simulink model "IndustrialMicrogrid"  (R2023a)
settings: Solver=FixedStepDiscrete  StartTime=0.0  StopTime=10  FixedStep=Ts  RelTol=1e-3
PostLoadFcn:
  | IndustrialMicrogridInputData
  | GfmGridFormingConverterInputParameters
model workspace (MAT data in the model file):
  caseNum = 2
undefined symbols (not defined in the file): base, BESS, DiscIntNeverNeededParam, grid, Grid, gridInverter, machine, microgrid, PV, PVInverter, PVTransformer, scrFactorRg, scrFactorXg, transformer, Ts
libraries: ee_lib x112, eeGeneralControl x104, nesl_utility_internal x64, simulink x56, nesl_utility x37, fl_lib x29, slpidlib x13, eeTransforms x11, eeTotalHarmonicDistorsion x8, eeRmsMeasurement x4, eeSinusoidalMeasurement x4, simulink_extras x2
(part 7 of 14)

== system IndustrialMicrogrid/MG1 Primary Substation/Microgrid Controller/Planned Island/Control for Zero Powerflow ==
  Bus Element In{,1..4} (5 alike) : Inport  PortName=ControlRoom  Element=PlannedIslandCmd
  In Bus Element1 : Inport  Port=2  PortName=mPCCPLL  Element=PCC.mPCC.reactivepower
  In Bus Element7 : Inport  Port=2  PortName=mPCCPLL  Element=PCC.mPCC.activepower
  Logical Operator : Logic  AllPortsSameDT=off  OutDataTypeStr=boolean
  PID Frequency : slpidlib/PID Controller  Controller=PI  Form=Parallel  TimeDomain=Discrete-time  UseExternalTs=off  SampleTime=2*Ts  IntegratorMethod=Forward Euler  FilterMethod=Forward Euler  ControllerParametersSource=internal  P=KpPPlannedIsland  I=KiPPlannedIsland  UseKiTs=off  D=0  N=100  UseFilter=on  TunerSelectOption=Frequency Response Based  InitialConditionSource=internal  InitialConditionForIntegrator=0  InitialConditionForFilter=0  DifferentiatorICPrevScaledInput=0  ExternalReset=none  TrackingMode=off  Kt=1  LimitOutput=off  SatLimitsSource=internal  UpperSaturationLimit=0.05  LowerSaturationLimit=-0.05  LinearizeAsGain=on  AntiWindupMode=clamping  Kb=1  LimitIntegrator=off  UpperIntegratorSaturationLimit=inf  LowerIntegratorSaturationLimit=-inf  POutMin=[]  POutMax=[]  IOutMin=[]  IOutMax=[]  DOutMin=[]  DOutMax=[]  NOutMin=[]  NOutMax=[]  SumOutMin=[]  SumOutMax=[]  SaturationOutMin=[]  SaturationOutMax=[]  PParamMin=[]  PParamMax=[]  IParamMin=[]  IParamMax=[]  DParamMin=[]  DParamMax=[]  NParamMin=[]  NParamMax=[]  KbParamMin=[]  KbParamMax=[]  KtParamMin=[]  KtParamMax=[]  KbOutMin=[]  KbOutMax=[]  KtOutMin=[]  KtOutMax=[]  IntegratorOutMin=[]  IntegratorOutMax=[]  FilterOutMin=[]  FilterOutMax=[]  SumI1OutMin=[]  SumI1OutMax=[]  SumI2OutMin=[]  SumI2OutMax=[]  SumI3OutMin=[]  SumI3OutMax=[]  SumI4OutMin=[]  SumI4OutMax=[]  SumDOutMin=[]  SumDOutMax=[]  DifferentiatorOutMin=[]  DifferentiatorOutMax=[]  FilterDiffOutCoefMin=[]  FilterDiffOutCoefMax=[]  ReciprocalOutMin=[]  ReciprocalOutMax=[]  SumDenOutMin=[]  SumDenOutMax=[]  SumNumOutMin=[]  SumNumOutMax=[]  DivideOutMin=[]  DivideOutMax=[]  UdiffTsProdOutMin=[]  UdiffTsProdOutMax=[]  NTsProdOutMin=[]  NTsProdOutMax=[]  UintegralTsProdOutMin=[]  UintegralTsProdOutMax=[]  UngainTsProdOutMin=[]  UngainTsProdOutMax=[]  ClampingZeroOutDataTypeStr=Inherit: Inherit via back propagation  ClampingZeroOutMin=[]  ClampingZeroOutMax=[]  FilterDenConstantOutDataTypeStr=Inherit: Inherit via back propagation  FilterDenConstantOutMin=[]  FilterDenConstantOutMax=[]  PCopyOutDataTypeStr=Inherit: Inherit via back propagation  PCopyOutMin=[]  PCopyOutMax=[]  NCopyOutDataTypeStr=Inherit: Inherit via back propagation  NCopyOutMin=[]  NCopyOutMax=[]  IntegratorContinuousStateAttributes=''  IntegratorStateMustResolveToSignalObject=off  IntegratorRTWStateStorageClass=Auto  FilterContinuousStateAttributes=''  FilterStateMustResolveToSignalObject=off  FilterRTWStateStorageClass=Auto  ParallelPVariant=InternalParameters  IdealPVariant=Disabled  IVariant=InternalParameters  DVariant=Disabled  IntegratorVariant=Discrete  SatVariant=Disabled  AWVariant=Passthrough  PCopyVariant=Disabled  TRVariant=Disabled  FdbkBlocksVariant=Forward  IdealPFdbkVariant=Disabled  SatFdbkVariant=Disabled  DerivativeFilterVariant=Disabled  NVariant=Disabled  NCopyVariant=Disabled_SignalSpec  FilterICVariant=Disabled  IntegratorICVariant=InternalICs  ExternalResetVariant=Disabled  TRSumVariant=Passthrough  SumFdbkVariant=Disabled  SumVariant=Sum_PI  TsampFilterVariant=InternalTs  TsampNgainVariant=Passthrough  TsampIntegralVariant=Disabled_SignalSpec  ExternalSaturationOutDataTypeStr=Inherit: Same as second input
  PID voltage : slpidlib/PID Controller  Controller=PI  Form=Parallel  TimeDomain=Discrete-time  UseExternalTs=off  SampleTime=2*Ts  IntegratorMethod=Forward Euler  FilterMethod=Forward Euler  ControllerParametersSource=internal  P=KpQPlannedIsland  I=KiQPlannedIsland  UseKiTs=off  D=0  N=100  UseFilter=on  TunerSelectOption=Frequency Response Based  InitialConditionSource=internal  InitialConditionForIntegrator=0  InitialConditionForFilter=0  DifferentiatorICPrevScaledInput=0  ExternalReset=none  TrackingMode=off  Kt=1  LimitOutput=off  SatLimitsSource=internal  UpperSaturationLimit=0.05  LowerSaturationLimit=-0.05  LinearizeAsGain=on  AntiWindupMode=clamping  Kb=1  LimitIntegrator=off  UpperIntegratorSaturationLimit=inf  LowerIntegratorSaturationLimit=-inf  POutMin=[]  POutMax=[]  IOutMin=[]  IOutMax=[]  DOutMin=[]  DOutMax=[]  NOutMin=[]  NOutMax=[]  SumOutMin=[]  SumOutMax=[]  SaturationOutMin=[]  SaturationOutMax=[]  PParamMin=[]  PParamMax=[]  IParamMin=[]  IParamMax=[]  DParamMin=[]  DParamMax=[]  NParamMin=[]  NParamMax=[]  KbParamMin=[]  KbParamMax=[]  KtParamMin=[]  KtParamMax=[]  KbOutMin=[]  KbOutMax=[]  KtOutMin=[]  KtOutMax=[]  IntegratorOutMin=[]  IntegratorOutMax=[]  FilterOutMin=[]  FilterOutMax=[]  SumI1OutMin=[]  SumI1OutMax=[]  SumI2OutMin=[]  SumI2OutMax=[]  SumI3OutMin=[]  SumI3OutMax=[]  SumI4OutMin=[]  SumI4OutMax=[]  SumDOutMin=[]  SumDOutMax=[]  DifferentiatorOutMin=[]  DifferentiatorOutMax=[]  FilterDiffOutCoefMin=[]  FilterDiffOutCoefMax=[]  ReciprocalOutMin=[]  ReciprocalOutMax=[]  SumDenOutMin=[]  SumDenOutMax=[]  SumNumOutMin=[]  SumNumOutMax=[]  DivideOutMin=[]  DivideOutMax=[]  UdiffTsProdOutMin=[]  UdiffTsProdOutMax=[]  NTsProdOutMin=[]  NTsProdOutMax=[]  UintegralTsProdOutMin=[]  UintegralTsProdOutMax=[]  UngainTsProdOutMin=[]  UngainTsProdOutMax=[]  ClampingZeroOutDataTypeStr=Inherit: Inherit via back propagation  ClampingZeroOutMin=[]  ClampingZeroOutMax=[]  FilterDenConstantOutDataTypeStr=Inherit: Inherit via back propagation  FilterDenConstantOutMin=[]  FilterDenConstantOutMax=[]  PCopyOutDataTypeStr=Inherit: Inherit via back propagation  PCopyOutMin=[]  PCopyOutMax=[]  NCopyOutDataTypeStr=Inherit: Inherit via back propagation  NCopyOutMin=[]  NCopyOutMax=[]  IntegratorContinuousStateAttributes=''  IntegratorStateMustResolveToSignalObject=off  IntegratorRTWStateStorageClass=Auto  FilterContinuousStateAttributes=''  FilterStateMustResolveToSignalObject=off  FilterRTWStateStorageClass=Auto  ParallelPVariant=InternalParameters  IdealPVariant=Disabled  IVariant=InternalParameters  DVariant=Disabled  IntegratorVariant=Discrete  SatVariant=Disabled  AWVariant=Passthrough  PCopyVariant=Disabled  TRVariant=Disabled  FdbkBlocksVariant=Forward  IdealPFdbkVariant=Disabled  SatFdbkVariant=Disabled  DerivativeFilterVariant=Disabled  NVariant=Disabled  NCopyVariant=Disabled_SignalSpec  FilterICVariant=Disabled  IntegratorICVariant=InternalICs  ExternalResetVariant=Disabled  TRSumVariant=Passthrough  SumFdbkVariant=Disabled  SumVariant=Sum_PI  TsampFilterVariant=InternalTs  TsampNgainVariant=Passthrough  TsampIntegralVariant=Disabled_SignalSpec  ExternalSaturationOutDataTypeStr=Inherit: Same as second input
  Planned Island Time Delay : Subsystem
  Product{,1..3} (4 alike) : Product
  Subsystem : Subsystem
  Subsystem1 : Subsystem
  Bus Element Out : Outport  PortName=MGController  Element=plannedisland
  Bus Element Out1 : Outport  PortName=MGController  Element=plannedislandP
  Bus Element Out2 : Outport  PortName=MGController  Element=plannedislandQ
  Bus Element Out4 : Outport  PortName=MGController  Element=activepowererror
  Bus Element Out6 : Outport  PortName=MGController  Element=reactivepowerrror
  wires:
  Logical Operator/1 -> Planned Island Time Delay/1(In1)
  Planned Island Time Delay/1(MGController) -> Bus Element Out/1
  Bus Element In3/1 -> Planned Island Time Delay/2(In2)
  PID voltage/1 -> Bus Element Out2/1  "REACTIVE POWER"
  Bus Element In2/1 -> Product2/2
  Bus Element In/1 -> Product1/2
  Product2/1 -> Subsystem1/1(REACTIVEPOWER ERROR), PID voltage/1, Bus Element Out6/1  "REACTIVEPOWER ERROR"
  Product1/1 -> PID Frequency/1, Bus Element Out4/1, Subsystem/1(AVTIVE POWER ERROR)  "AVTIVE POWER ERROR"
  PID Frequency/1 -> Bus Element Out1/1  "ACTIVE POWER"
  In Bus Element1/1 -> Product2/1
  In Bus Element7/1 -> Product1/1
  Bus Element In1/1 -> Product/1
  Product/1 -> Logical Operator/1
  Product3/1 -> Logical Operator/2
  Bus Element In4/1 -> Product3/1
  Subsystem/1(Out1) -> Product/2
  Subsystem1/1(Out1) -> Product3/2

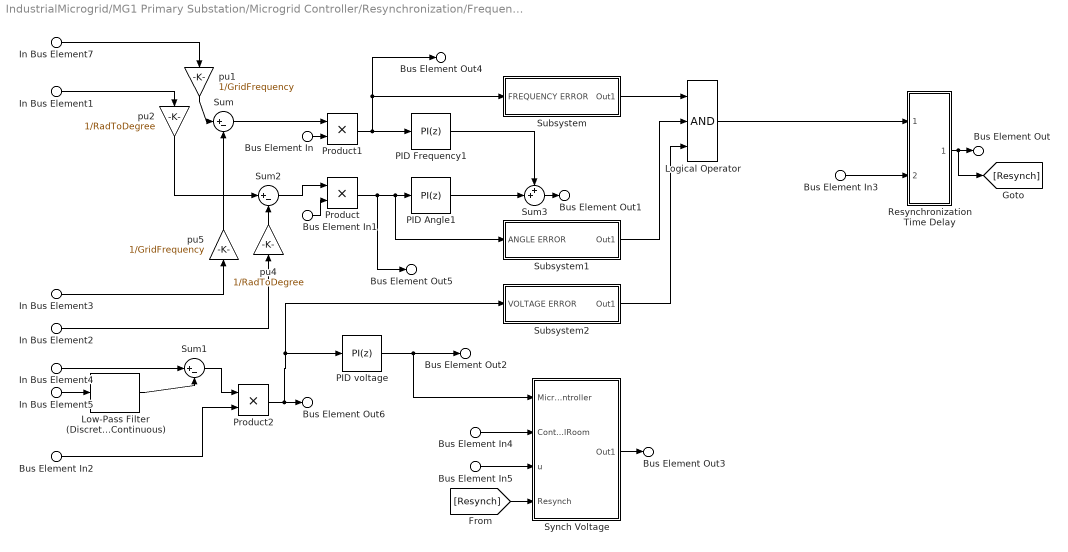
== system IndustrialMicrogrid/MG1 Primary Substation/Microgrid Controller/Resynchronization/Frequency and voltage matching ==
  Bus Element In5 : Inport  PortName=BESS  Element=reactive power
  Bus Element In{,1..4} (5 alike) : Inport  Port=2  PortName=ControlRoom  Element=ResynchCmd
  In Bus Element1 : Inport  Port=3  PortName=mPCCPLL  Element=Grid.angle
  In Bus Element7 : Inport  Port=3  PortName=mPCCPLL  Element=Grid.frequency
  In Bus Element4 : Inport  Port=3  PortName=mPCCPLL  Element=Grid.voltage
  In Bus Element3 : Inport  Port=3  PortName=mPCCPLL  Element=Island.frequency
  In Bus Element2 : Inport  Port=3  PortName=mPCCPLL  Element=Island.angle
  In Bus Element5 : Inport  Port=3  PortName=mPCCPLL  Element=Island.voltage
  Logical Operator : Logic  Inputs=3  AllPortsSameDT=off  OutDataTypeStr=boolean
  Low-Pass Filter (Discrete or Continuous) : eeGeneralControl/Low-Pass Filter (Discrete or Continuous)  K=1  T=0.04  B=inf  A=-inf  init_option=Inherited from block input  x0=0  Ts=-1
  PID Angle1 : slpidlib/PID Controller  Controller=PI  Form=Parallel  TimeDomain=Discrete-time  UseExternalTs=off  SampleTime=2*Ts  IntegratorMethod=Forward Euler  FilterMethod=Forward Euler  ControllerParametersSource=internal  P=KpAngResynch  I=KiAngResynch  UseKiTs=off  D=0  N=100  UseFilter=on  TunerSelectOption=Frequency Response Based  InitialConditionSource=internal  InitialConditionForIntegrator=0  InitialConditionForFilter=0  DifferentiatorICPrevScaledInput=0  ExternalReset=none  TrackingMode=off  Kt=1  LimitOutput=off  SatLimitsSource=internal  UpperSaturationLimit=0.05  LowerSaturationLimit=-0.05  LinearizeAsGain=on  AntiWindupMode=clamping  Kb=1  LimitIntegrator=off  UpperIntegratorSaturationLimit=inf  LowerIntegratorSaturationLimit=-inf  POutMin=[]  POutMax=[]  IOutMin=[]  IOutMax=[]  DOutMin=[]  DOutMax=[]  NOutMin=[]  NOutMax=[]  SumOutMin=[]  SumOutMax=[]  SaturationOutMin=[]  SaturationOutMax=[]  PParamMin=[]  PParamMax=[]  IParamMin=[]  IParamMax=[]  DParamMin=[]  DParamMax=[]  NParamMin=[]  NParamMax=[]  KbParamMin=[]  KbParamMax=[]  KtParamMin=[]  KtParamMax=[]  KbOutMin=[]  KbOutMax=[]  KtOutMin=[]  KtOutMax=[]  IntegratorOutMin=[]  IntegratorOutMax=[]  FilterOutMin=[]  FilterOutMax=[]  SumI1OutMin=[]  SumI1OutMax=[]  SumI2OutMin=[]  SumI2OutMax=[]  SumI3OutMin=[]  SumI3OutMax=[]  SumI4OutMin=[]  SumI4OutMax=[]  SumDOutMin=[]  SumDOutMax=[]  DifferentiatorOutMin=[]  DifferentiatorOutMax=[]  FilterDiffOutCoefMin=[]  FilterDiffOutCoefMax=[]  ReciprocalOutMin=[]  ReciprocalOutMax=[]  SumDenOutMin=[]  SumDenOutMax=[]  SumNumOutMin=[]  SumNumOutMax=[]  DivideOutMin=[]  DivideOutMax=[]  UdiffTsProdOutMin=[]  UdiffTsProdOutMax=[]  NTsProdOutMin=[]  NTsProdOutMax=[]  UintegralTsProdOutMin=[]  UintegralTsProdOutMax=[]  UngainTsProdOutMin=[]  UngainTsProdOutMax=[]  ClampingZeroOutDataTypeStr=Inherit: Inherit via back propagation  ClampingZeroOutMin=[]  ClampingZeroOutMax=[]  FilterDenConstantOutDataTypeStr=Inherit: Inherit via back propagation  FilterDenConstantOutMin=[]  FilterDenConstantOutMax=[]  PCopyOutDataTypeStr=Inherit: Inherit via back propagation  PCopyOutMin=[]  PCopyOutMax=[]  NCopyOutDataTypeStr=Inherit: Inherit via back propagation  NCopyOutMin=[]  NCopyOutMax=[]  IntegratorContinuousStateAttributes=''  IntegratorStateMustResolveToSignalObject=off  IntegratorRTWStateStorageClass=Auto  FilterContinuousStateAttributes=''  FilterStateMustResolveToSignalObject=off  FilterRTWStateStorageClass=Auto  ParallelPVariant=InternalParameters  IdealPVariant=Disabled  IVariant=InternalParameters  DVariant=Disabled  IntegratorVariant=Discrete  SatVariant=Disabled  AWVariant=Passthrough  PCopyVariant=Disabled  TRVariant=Disabled  FdbkBlocksVariant=Forward  IdealPFdbkVariant=Disabled  SatFdbkVariant=Disabled  DerivativeFilterVariant=Disabled  NVariant=Disabled  NCopyVariant=Disabled_SignalSpec  FilterICVariant=Disabled  IntegratorICVariant=InternalICs  ExternalResetVariant=Disabled  TRSumVariant=Passthrough  SumFdbkVariant=Disabled  SumVariant=Sum_PI  TsampFilterVariant=InternalTs  TsampNgainVariant=Passthrough  TsampIntegralVariant=Disabled_SignalSpec  ExternalSaturationOutDataTypeStr=Inherit: Same as second input
  PID Frequency1 : slpidlib/PID Controller  Controller=PI  Form=Parallel  TimeDomain=Discrete-time  UseExternalTs=off  SampleTime=2*Ts  IntegratorMethod=Forward Euler  FilterMethod=Forward Euler  ControllerParametersSource=internal  P=KpFreResynch  I=KiFreResynch  UseKiTs=off  D=0  N=100  UseFilter=on  TunerSelectOption=Frequency Response Based  InitialConditionSource=internal  InitialConditionForIntegrator=0  InitialConditionForFilter=0  DifferentiatorICPrevScaledInput=0  ExternalReset=none  TrackingMode=off  Kt=1  LimitOutput=off  SatLimitsSource=internal  UpperSaturationLimit=0.05  LowerSaturationLimit=-0.05  LinearizeAsGain=on  AntiWindupMode=clamping  Kb=1  LimitIntegrator=off  UpperIntegratorSaturationLimit=inf  LowerIntegratorSaturationLimit=-inf  POutMin=[]  POutMax=[]  IOutMin=[]  IOutMax=[]  DOutMin=[]  DOutMax=[]  NOutMin=[]  NOutMax=[]  SumOutMin=[]  SumOutMax=[]  SaturationOutMin=[]  SaturationOutMax=[]  PParamMin=[]  PParamMax=[]  IParamMin=[]  IParamMax=[]  DParamMin=[]  DParamMax=[]  NParamMin=[]  NParamMax=[]  KbParamMin=[]  KbParamMax=[]  KtParamMin=[]  KtParamMax=[]  KbOutMin=[]  KbOutMax=[]  KtOutMin=[]  KtOutMax=[]  IntegratorOutMin=[]  IntegratorOutMax=[]  FilterOutMin=[]  FilterOutMax=[]  SumI1OutMin=[]  SumI1OutMax=[]  SumI2OutMin=[]  SumI2OutMax=[]  SumI3OutMin=[]  SumI3OutMax=[]  SumI4OutMin=[]  SumI4OutMax=[]  SumDOutMin=[]  SumDOutMax=[]  DifferentiatorOutMin=[]  DifferentiatorOutMax=[]  FilterDiffOutCoefMin=[]  FilterDiffOutCoefMax=[]  ReciprocalOutMin=[]  ReciprocalOutMax=[]  SumDenOutMin=[]  SumDenOutMax=[]  SumNumOutMin=[]  SumNumOutMax=[]  DivideOutMin=[]  DivideOutMax=[]  UdiffTsProdOutMin=[]  UdiffTsProdOutMax=[]  NTsProdOutMin=[]  NTsProdOutMax=[]  UintegralTsProdOutMin=[]  UintegralTsProdOutMax=[]  UngainTsProdOutMin=[]  UngainTsProdOutMax=[]  ClampingZeroOutDataTypeStr=Inherit: Inherit via back propagation  ClampingZeroOutMin=[]  ClampingZeroOutMax=[]  FilterDenConstantOutDataTypeStr=Inherit: Inherit via back propagation  FilterDenConstantOutMin=[]  FilterDenConstantOutMax=[]  PCopyOutDataTypeStr=Inherit: Inherit via back propagation  PCopyOutMin=[]  PCopyOutMax=[]  NCopyOutDataTypeStr=Inherit: Inherit via back propagation  NCopyOutMin=[]  NCopyOutMax=[]  IntegratorContinuousStateAttributes=''  IntegratorStateMustResolveToSignalObject=off  IntegratorRTWStateStorageClass=Auto  FilterContinuousStateAttributes=''  FilterStateMustResolveToSignalObject=off  FilterRTWStateStorageClass=Auto  ParallelPVariant=InternalParameters  IdealPVariant=Disabled  IVariant=InternalParameters  DVariant=Disabled  IntegratorVariant=Discrete  SatVariant=Disabled  AWVariant=Passthrough  PCopyVariant=Disabled  TRVariant=Disabled  FdbkBlocksVariant=Forward  IdealPFdbkVariant=Disabled  SatFdbkVariant=Disabled  DerivativeFilterVariant=Disabled  NVariant=Disabled  NCopyVariant=Disabled_SignalSpec  FilterICVariant=Disabled  IntegratorICVariant=InternalICs  ExternalResetVariant=Disabled  TRSumVariant=Passthrough  SumFdbkVariant=Disabled  SumVariant=Sum_PI  TsampFilterVariant=InternalTs  TsampNgainVariant=Passthrough  TsampIntegralVariant=Disabled_SignalSpec  ExternalSaturationOutDataTypeStr=Inherit: Same as second input
  PID voltage : slpidlib/PID Controller  Controller=PI  Form=Parallel  TimeDomain=Discrete-time  UseExternalTs=off  SampleTime=2*Ts  IntegratorMethod=Forward Euler  FilterMethod=Forward Euler  ControllerParametersSource=internal  P=KpVolResynch  I=KiVolResynch  UseKiTs=off  D=0  N=100  UseFilter=on  TunerSelectOption=Frequency Response Based  InitialConditionSource=internal  InitialConditionForIntegrator=1  InitialConditionForFilter=0  DifferentiatorICPrevScaledInput=0  ExternalReset=none  TrackingMode=off  Kt=1  LimitOutput=off  SatLimitsSource=internal  UpperSaturationLimit=0.05  LowerSaturationLimit=-0.05  LinearizeAsGain=on  AntiWindupMode=clamping  Kb=1  LimitIntegrator=off  UpperIntegratorSaturationLimit=inf  LowerIntegratorSaturationLimit=-inf  POutMin=[]  POutMax=[]  IOutMin=[]  IOutMax=[]  DOutMin=[]  DOutMax=[]  NOutMin=[]  NOutMax=[]  SumOutMin=[]  SumOutMax=[]  SaturationOutMin=[]  SaturationOutMax=[]  PParamMin=[]  PParamMax=[]  IParamMin=[]  IParamMax=[]  DParamMin=[]  DParamMax=[]  NParamMin=[]  NParamMax=[]  KbParamMin=[]  KbParamMax=[]  KtParamMin=[]  KtParamMax=[]  KbOutMin=[]  KbOutMax=[]  KtOutMin=[]  KtOutMax=[]  IntegratorOutMin=[]  IntegratorOutMax=[]  FilterOutMin=[]  FilterOutMax=[]  SumI1OutMin=[]  SumI1OutMax=[]  SumI2OutMin=[]  SumI2OutMax=[]  SumI3OutMin=[]  SumI3OutMax=[]  SumI4OutMin=[]  SumI4OutMax=[]  SumDOutMin=[]  SumDOutMax=[]  DifferentiatorOutMin=[]  DifferentiatorOutMax=[]  FilterDiffOutCoefMin=[]  FilterDiffOutCoefMax=[]  ReciprocalOutMin=[]  ReciprocalOutMax=[]  SumDenOutMin=[]  SumDenOutMax=[]  SumNumOutMin=[]  SumNumOutMax=[]  DivideOutMin=[]  DivideOutMax=[]  UdiffTsProdOutMin=[]  UdiffTsProdOutMax=[]  NTsProdOutMin=[]  NTsProdOutMax=[]  UintegralTsProdOutMin=[]  UintegralTsProdOutMax=[]  UngainTsProdOutMin=[]  UngainTsProdOutMax=[]  ClampingZeroOutDataTypeStr=Inherit: Inherit via back propagation  ClampingZeroOutMin=[]  ClampingZeroOutMax=[]  FilterDenConstantOutDataTypeStr=Inherit: Inherit via back propagation  FilterDenConstantOutMin=[]  FilterDenConstantOutMax=[]  PCopyOutDataTypeStr=Inherit: Inherit via back propagation  PCopyOutMin=[]  PCopyOutMax=[]  NCopyOutDataTypeStr=Inherit: Inherit via back propagation  NCopyOutMin=[]  NCopyOutMax=[]  IntegratorContinuousStateAttributes=''  IntegratorStateMustResolveToSignalObject=off  IntegratorRTWStateStorageClass=Auto  FilterContinuousStateAttributes=''  FilterStateMustResolveToSignalObject=off  FilterRTWStateStorageClass=Auto  ParallelPVariant=InternalParameters  IdealPVariant=Disabled  IVariant=InternalParameters  DVariant=Disabled  IntegratorVariant=Discrete  SatVariant=Disabled  AWVariant=Passthrough  PCopyVariant=Disabled  TRVariant=Disabled  FdbkBlocksVariant=Forward  IdealPFdbkVariant=Disabled  SatFdbkVariant=Disabled  DerivativeFilterVariant=Disabled  NVariant=Disabled  NCopyVariant=Disabled_SignalSpec  FilterICVariant=Disabled  IntegratorICVariant=InternalICs  ExternalResetVariant=Disabled  TRSumVariant=Passthrough  SumFdbkVariant=Disabled  SumVariant=Sum_PI  TsampFilterVariant=InternalTs  TsampNgainVariant=Passthrough  TsampIntegralVariant=Disabled_SignalSpec  ExternalSaturationOutDataTypeStr=Inherit: Same as second input
  Product : Product
  Product1 : Product
  Product2 : Product
  Resynchronization Time Delay : Subsystem
  Subsystem : Subsystem
  Subsystem1 : Subsystem
  Subsystem2 : Subsystem
  Sum : Sum  Inputs=|+-
  Sum1 : Sum  Inputs=|+-
  Sum2 : Sum  Inputs=|+-
  Sum3 : Sum  Inputs=++|
  Synch Voltage : Subsystem
  pu1 : Gain  Gain=1/GridFrequency
  pu2 : Gain  Gain=1/RadToDegree
  pu4 : Gain  Gain=1/RadToDegree
  pu5 : Gain  Gain=1/GridFrequency
  Bus Element Out : Outport  PortName=MGController  Element=resynch
  Bus Element Out1 : Outport  PortName=MGController  Element=synchfrequency
  Bus Element Out2 : Outport  PortName=MGController  Element=synchvoltage
  Bus Element Out3 : Outport  PortName=MGController  Element=synchvoltagedpr
  Bus Element Out4 : Outport  PortName=MGController  Element=frequencyerror
  Bus Element Out5 : Outport  PortName=MGController  Element=phaseerror
  Bus Element Out6 : Outport  PortName=MGController  Element=voltagemagerror
  wires:
  Sum/1 -> Product1/1
  pu1/1 -> Sum/1
  pu4/1 -> Sum2/2
  pu2/1 -> Sum2/1
  pu5/1 -> Sum/2
  In Bus Element2/1 -> pu4/1
  In Bus Element3/1 -> pu5/1
  Sum1/1 -> Product2/1
  Subsystem/1(Out1) -> Logical Operator/1
  Subsystem1/1(Out1) -> Logical Operator/2
  Subsystem2/1(Out1) -> Logical Operator/3
  Sum3/1 -> Bus Element Out1/1
  PID Frequency1/1 -> Sum3/1
  PID Angle1/1 -> Sum3/2
  Sum2/1 -> Product/1
  Product/1 -> Bus Element Out5/1, Subsystem1/1(ANGLE ERROR), PID Angle1/1
  Product1/1 -> Bus Element Out4/1, Subsystem/1(FREQUENCY ERROR), PID Frequency1/1
  Product2/1 -> Subsystem2/1(VOLTAGE ERROR), PID voltage/1, Bus Element Out6/1
  Bus Element In/1 -> Product1/2
  Bus Element In1/1 -> Product/2
  Bus Element In2/1 -> Product2/2
  In Bus Element7/1 -> pu1/1
  In Bus Element1/1 -> pu2/1
  In Bus Element4/1 -> Sum1/1
  In Bus Element5/1 -> Low-Pass Filter (Discrete or Continuous)/1
  PID voltage/1 -> Bus Element Out2/1, Synch Voltage/1(MicrogridController)
  Bus Element In3/1 -> Resynchronization Time Delay/2(In2)
  Resynchronization Time Delay/1(MGController) -> [Resynch], Bus Element Out/1
  Logical Operator/1 -> Resynchronization Time Delay/1(In1)
  Bus Element In4/1 -> Synch Voltage/2(ControlRoom)
  Bus Element In5/1 -> Synch Voltage/3(u)
  Synch Voltage/1(Out1) -> Bus Element Out3/1
  [Resynch] -> Synch Voltage/4(Resynch)
  Low-Pass Filter (Discrete or Continuous)/1 -> Sum1/2

== system IndustrialMicrogrid/MG2 PV Plant/(500KWp PV)/PV Inverter A2/PV & Inverter ==
  note: Calculated PV power output
  note: Measured PV current
  note: Perturb & Observe method for maximum power point (MPP) tracking of PV array
  note: DC bus voltage reference (which is the MPP voltage)
  Solar insolation : Inport
  reference : Inport  Port=2
  Average-Inverter : ee_lib/Semiconductors & Converters/Converters/Average-Value Voltage Source Converter (Three-Phase)  port_option=ee.enum.threePhasePort.composite  frequency_option=ee.enum.converters.frequency.variable  FRated=60 Hz  losses_parameterization=ee.enum.converters.losses.fixed  Pfixed=1 W  ks=0.01  kc1=1.7 V  kc2=0.01 Ohm  Ploss_vect=[100, 800, 1870, 3250, 4900] W  Irms_vect=[10, 100, 200, 300, 400] A  Vdc_nom=300 V  thermal_mass=30000 J/K  temperature_specify=off  temperature_priority=High  temperature=298.15 K  temperature_nominal_specify=off  temperature_nominal_unit=K  temperature_nominal_value=1
      settings: InternalSimscapePortConfiguration="{\"Bottom\":[],\"Left\":[{\"id\":\"ModWave\",\"label\":\"ModWave\",\"type\":\"input\"},{\"id\":\"N\",\"label\":\"~\",\"type\":\"foundation.electrical.three_phase\"}],\"Right\":[{\"id\":\"p\",\"label\":\"+\",\"type\":\"foundation.electrical.electrical\"},{\"id\":\"n\",\"label\":\"-\",\"type\":\"foundation.electrical.electrical\"}],\"Top\":[]}"
  Current Sensor : fl_lib/Electrical/Electrical Sensors/Current Sensor
  DC- Capacitor : fl_lib/Electrical/Electrical Elements/Capacitor  c=PVInverter.c F  r=1e-6 Ohm  g=0 1/Ohm  i_specify=off  i_priority=None  i=0 A  i_nominal_specify=off  i_nominal_unit=A  i_nominal_value=1  v_specify=off  v_priority=None  v=6560*.5 V  v_nominal_specify=off  v_nominal_unit=V  v_nominal_value=1  vc_specify=on  vc_priority=None  vc=PVInverter.Vdc V  vc_nominal_specify=off  vc_nominal_unit=V  vc_nominal_value=1
  ERef1 : fl_lib/Electrical/Electrical Elements/Electrical Reference
  Low-Pass Filter (Discrete or Continuous) : eeGeneralControl/Low-Pass Filter (Discrete or Continuous)  K=1  T=0.2  B=inf  A=-inf  init_option=Inherited from block input  x0=0  Ts=-1
  Low-Pass Filter (Discrete or Continuous)1 : eeGeneralControl/Low-Pass Filter (Discrete or Continuous)  K=1  T=0.2  B=inf  A=-inf  init_option=Inherited from block input  x0=0  Ts=-1
  Measurement1 : Subsystem
  Measurement2 : Subsystem
  P&O MPP : Subsystem
  PS-Simulink Converter : nesl_utility/PS-Simulink Converter  PhysicalDomain=network_engine_domain  SubClassName=ps_output  LeftPortType=input  RightPortType=output  PseudoPeriodic=off  Frequencies=[]  VectorFormat=inherit  Unit=inherit  AffineConversion=off
  PS-Simulink Converter1 : nesl_utility/PS-Simulink Converter  PhysicalDomain=network_engine_domain  SubClassName=ps_output  LeftPortType=input  RightPortType=output  PseudoPeriodic=off  Frequencies=[]  VectorFormat=inherit  Unit=inherit  AffineConversion=off
  PV Array : ee_lib/Sources/Solar Cell  prm=3  Isc=3.8 A  Voc=0.586 V  Is=PV.solarCellDiodeSaturationCurrent A  Is2=0 A  Iph=PV.solarCellSolarGeneratedCurrentAM A  Ir0=1000 W/m^2  ec=PV.solarCellQualityFactorI  N2=PV.solarCellQualityFactorJ  Rs=PV.solarCellSeriesResistance Ohm  Rp=PV.solarCellParallelResistance Ohm  N_series=PV.panelNSeriesCellPanel*PV.arrayNseriesPanelsPerString  N_parallel=PV.PanelNParallelStringsPanel*PV.arrayNParallelStrings  TIPH1=PV.solarCellTempCofficient 1/K  EG=PV.solarCellEg eV  TXIS1=PV.solarCellTemparatureExponentIs1  TXIS2=PV.solarCellTemparatureExponentIs2  TRS1=PV.solarCellTemparatureExponentRs  TRP1=PV.solarCellTemparatureExponentRp  Tmeas=PV.solarCellMeasurementTemperature degC  TFIXED=PV.solarCellDeviceTemperature degC  thermal_mass=100 J/K  initial_temperature=25 degC
  Product2 : Product
  Simulink-PS Converter1 : nesl_utility/Simulink-PS Converter  PhysicalDomain=network_engine_domain  SubClassName=ps_input  LeftPortType=input  RightPortType=output  PseudoPeriodic=off  Frequencies=[]  NoiseDistribution=none  NoiseParameters=[]  Unit=1  AffineConversion=off  FilteringAndDerivatives=provide  SimscapeFilterOrder=1  InputFilterTimeConstant=0.001  UdotUserProvided=0
  Simulink-PS Converter2 : nesl_utility/Simulink-PS Converter  PhysicalDomain=network_engine_domain  SubClassName=ps_input  LeftPortType=input  RightPortType=output  PseudoPeriodic=off  Frequencies=[]  NoiseDistribution=none  NoiseParameters=[]  Unit=1  AffineConversion=off  FilteringAndDerivatives=provide  SimscapeFilterOrder=1  InputFilterTimeConstant=0.001  UdotUserProvided=0
  Voltage Sensor : fl_lib/Electrical/Electrical Sensors/Voltage Sensor
  Conn1 : PMIOPort  Side=Right
  Out Bus Element4 : Outport  PortName=PV_plant1  Element=Vdc_ref
  Out Bus Element : Outport  PortName=PV_plant1  Element=Pref1
  Out Bus Element3 : Outport  PortName=PV_plant1  Element=Vdc_measured
  Out Bus Element1 : Outport  PortName=PV_plant1  Element=ipv
  wires:
  Low-Pass Filter (Discrete or Continuous)1/1 -> Product2/2
  Low-Pass Filter (Discrete or Continuous)/1 -> [Vdc]
  Measurement2/1(Out1) -> [ipv]
  Measurement1/1(Out1) -> Low-Pass Filter (Discrete or Continuous)/1
  [Vdc] -> P&O MPP/2(Input)
  P&O MPP/1(Vmpp) -> Out Bus Element4/1
  Product2/1 -> Out Bus Element/1, P&O MPP/1(In1)
  reference/1 -> Simulink-PS Converter2/1
  [Vdc] -> Product2/1
  PS-Simulink Converter/1 -> Out Bus Element3/1, Measurement1/1(u)
  [ipv] -> Low-Pass Filter (Discrete or Continuous)1/1
  Solar insolation/1 -> Simulink-PS Converter1/1
  PS-Simulink Converter1/1 -> Out Bus Element1/1, Measurement2/1(u)
  connections:
  PV Array/RConn1 -- ERef1/LConn1 -- DC- Capacitor/RConn1 -- Average-Inverter/RConn2 -- Voltage Sensor/RConn2
  Simulink-PS Converter1/RConn1 -- PV Array/LConn1
  PS-Simulink Converter1/LConn1 -- Current Sensor/RConn1
  Conn1/RConn1 -- Average-Inverter/LConn2
  PV Array/LConn2 -- Current Sensor/LConn1
  Average-Inverter/LConn1 -- Simulink-PS Converter2/RConn1
  Voltage Sensor/LConn1 -- Current Sensor/RConn2 -- Average-Inverter/RConn1 -- DC- Capacitor/LConn1
  PS-Simulink Converter/LConn1 -- Voltage Sensor/RConn1

== system IndustrialMicrogrid/MG2 PV Plant/(500KWp PV)/PV Inverter A2/PV Controller ==
  note: DQ/abc Transformation
  In Bus Element17 : Inport  PortName=PV_plant1  Element=Pref1
  In Bus Element18 : Inport  PortName=PV_plant1  Element=Vdc_measured
  In Bus Element19 : Inport  PortName=PV_plant1  Element=Vdc_ref
  In Bus Element5 : Inport  Port=2  PortName=ipv1  Element=1
  In Bus Element4 : Inport  Port=3  PortName=LVRT
  In Bus Element3 : Inport  Port=4  PortName=Vbus  Element=Vd
  In Bus Element1 : Inport  Port=4  PortName=Vbus  Element=Vd
  In Bus Element2 : Inport  Port=4  PortName=Vbus  Element=Vq
  In Bus Element6 : Inport  Port=4  PortName=Vbus  Element=Theta
  In Bus Element7 : Inport  Port=4  PortName=Vbus  Element=Theta
  Q_ref : Inport  Port=5
  Current_controller : Subsystem
  DC voltage controller & current reference : Subsystem
  Demux1 : Demux  Outputs=3
  Inverse Park Transform1 : eeTransforms/Inverse Park Transform  AxisAlignment=Q-axis  PowerInvariant=off
  Park Transform1 : eeTransforms/Park Transform  AxisAlignment=Q-axis  PowerInvariant=off
  Terminator1 : Terminator
  Unit Delay2 : UnitDelay  SampleTime=Ts  HasFrameUpgradeWarning=on
  m_abc : Outport
  wires:
  Q_ref/1 -> DC voltage controller & current reference/1(Q_ref)
  DC voltage controller & current reference/2(id_ref) -> [id_ref]
  DC voltage controller & current reference/1(iq_ref) -> [iq_ref]
  In Bus Element19/1 -> DC voltage controller & current reference/5(PV_vdc)
  In Bus Element18/1 -> DC voltage controller & current reference/4(PV_Mpp_vdc)
  In Bus Element17/1 -> DC voltage controller & current reference/3(P_pv)
  In Bus Element4/1 -> DC voltage controller & current reference/6(LVRT.iq)
  In Bus Element1/1 -> DC voltage controller & current reference/2(Vmag)
  In Bus Element5/1 -> Park Transform1/1
  [ipvd] -> Current_controller/2(ipvd)
  In Bus Element7/1 -> Inverse Park Transform1/2
  In Bus Element6/1 -> Park Transform1/2
  [ipvq] -> Current_controller/4(iq)
  [iq_ref] -> Current_controller/3(iqref)
  In Bus Element3/1 -> Current_controller/5(Vd)
  [id_ref] -> Current_controller/1(id-ref)
  Park Transform1/1 -> Demux1/1
  [mdqo] -> Inverse Park Transform1/1
  Demux1/3 -> Terminator1/1
  Demux1/1 -> [ipvd]
  Unit Delay2/1 -> m_abc/1
  Demux1/2 -> [ipvq]
  Inverse Park Transform1/1 -> Unit Delay2/1
  Current_controller/1(Refrence_mdq0) -> [mdqo]
  In Bus Element2/1 -> Current_controller/6(Vq)

== system IndustrialMicrogrid/MG2 Power Center/Diesel Generator/Governor and Prime Mover /Governor ==
  pu_velocity : Inport
  1/T_G : Gain  Gain=1/T_G
  1/droop : Gain  Gain=1/(droop_percentage/100)
  Delta load setpoint : Sum  Inputs=+-|
  Delta speed : Sum  Inputs=-+|
  Discrete-Time Integrator1 : DiscreteIntegrator  InitialCondition=pu_torque0  SampleTime=-1  ICPrevOutput=DiscIntNeverNeededParam  ICPrevScaledInput=DiscIntNeverNeededParam
  Load_setpoint : Constant  Value=pu_load_reference_setpoint
  Speed_ref : Constant  Value=pu_speed_reference
  Subtract : Sum  Inputs=|+-
  delta_y : Outport  VectorParamsAs1DForOutWhenUnconnected=off
  wires:
  Speed_ref/1 -> Delta speed/1
  Delta speed/1 -> 1/droop/1
  Load_setpoint/1 -> Delta load setpoint/1
  pu_velocity/1 -> Delta speed/2
  1/droop/1 -> Delta load setpoint/2
  Delta load setpoint/1 -> Subtract/1
  Subtract/1 -> 1/T_G/1
  1/T_G/1 -> Discrete-Time Integrator1/1
  Discrete-Time Integrator1/1 -> delta_y/1, Subtract/2

== system IndustrialMicrogrid/MG2 Power Center/Diesel Generator/Governor and Prime Mover /Non-reheat turbine ==
  delta_y : Inport
  1/T_CH : Gain  Gain=1/T_CH
  Discrete-Time Integrator1 : DiscreteIntegrator  InitialCondition=pu_torque0  SampleTime=-1  ICPrevOutput=DiscIntNeverNeededParam  ICPrevScaledInput=DiscIntNeverNeededParam
  Sum : Sum  Inputs=|+-
  torque : Outport  VectorParamsAs1DForOutWhenUnconnected=off
  wires:
  delta_y/1 -> Sum/1
  Sum/1 -> 1/T_CH/1
  1/T_CH/1 -> Discrete-Time Integrator1/1
  Discrete-Time Integrator1/1 -> Sum/2, torque/1

== system IndustrialMicrogrid/MG2 Primary Substation/BESS and Controller 2/BESS/Filter & Sensor ==
  Current Sensor (Three-Phase) : ee_lib/Sensors & Transducers/Current Sensor (Three-Phase)
  Electrical Reference1 : fl_lib/Electrical/Electrical Elements/Electrical Reference
  Low-Pass Filter (Discrete or Continuous)1 : eeGeneralControl/Low-Pass Filter (Discrete or Continuous)  K=1  T=1/(200*gridInverter.frequency)  B=inf  A=-inf  init_option=Specify as parameter  x0=0  Ts=gridInverter.controller.VoltageControlSampleTime
  Low-Pass Filter (Discrete or Continuous)2 : eeGeneralControl/Low-Pass Filter (Discrete or Continuous)  K=1  T=1/(200*gridInverter.frequency)  B=inf  A=-inf  init_option=Specify as parameter  x0=0  Ts=gridInverter.controller.VoltageControlSampleTime
  Neutral Port (Three-Phase) : ee_lib/Connectors & References/Neutral Port (Three-Phase)  G_parasitic=1e-12 1/Ohm
      settings: InternalSimscapePortConfiguration="{\"Bottom\":[],\"Left\":[{\"id\":\"N\",\"label\":\"~\",\"type\":\"foundation.electrical.three_phase\"}],\"Right\":[{\"id\":\"n\",\"label\":\"n\",\"type\":\"foundation.electrical.electrical\"}],\"Top\":[]}"
  PS-Simulink Converter : nesl_utility/PS-Simulink Converter  PhysicalDomain=network_engine_domain  SubClassName=ps_output  LeftPortType=input  RightPortType=output  PseudoPeriodic=off  Frequencies=[]  VectorFormat=inherit  Unit=inherit  AffineConversion=off
  PS-Simulink Converter1 : nesl_utility/PS-Simulink Converter  PhysicalDomain=network_engine_domain  SubClassName=ps_output  LeftPortType=input  RightPortType=output  PseudoPeriodic=off  Frequencies=[]  VectorFormat=inherit  Unit=inherit  AffineConversion=off
  Phase Voltage Sensor (Three-Phase) : ee_lib/Sensors & Transducers/Phase Voltage Sensor (Three-Phase)
  RLC (Three-Phase) : ee_lib/Passive/RLC Assemblies/RLC (Three-Phase)  component_structure=ee.enum.rlc.structure.SeriesRL  R=gridInverter.lineResistance Ohm  L=gridInverter.L*10 H  C=1e-6 F  R_parasitic=0 Ohm  G_parasitic=0 1/Ohm  IL_specify=off  IL_priority=High  IL=[0, 0, 0] A  IL_nominal_specify=off  IL_nominal_unit=A  IL_nominal_value=1  VC_specify=off  VC_priority=High  VC=[0, 0, 0] V  VC_nominal_specify=off  VC_nominal_unit=V  VC_nominal_value=1
      settings: InternalSimscapePortConfiguration="{\"Bottom\":[],\"Left\":[{\"id\":\"N1\",\"label\":\"~1\",\"type\":\"foundation.electrical.three_phase\"}],\"Right\":[{\"id\":\"N2\",\"label\":\"~2\",\"type\":\"foundation.electrical.three_phase\"}],\"Top\":[]}"
  Inabc : PMIOPort  Side=Left
  Opabc : PMIOPort  Port=2  Side=Right
  Iabc : Outport
  Vabc : Outport  Port=2
  wires:
  PS-Simulink Converter1/1 -> Low-Pass Filter (Discrete or Continuous)1/1
  Low-Pass Filter (Discrete or Continuous)2/1 -> Iabc/1
  PS-Simulink Converter/1 -> Low-Pass Filter (Discrete or Continuous)2/1
  Low-Pass Filter (Discrete or Continuous)1/1 -> Vabc/1
  connections:
  Electrical Reference1/LConn1 -- Neutral Port (Three-Phase)/RConn1
  PS-Simulink Converter1/LConn1 -- Phase Voltage Sensor (Three-Phase)/RConn1
  Current Sensor (Three-Phase)/RConn2 -- RLC (Three-Phase)/LConn1
  Neutral Port (Three-Phase)/LConn1 -- Phase Voltage Sensor (Three-Phase)/RConn2
  Current Sensor (Three-Phase)/LConn1 -- Inabc/RConn1
  PS-Simulink Converter/LConn1 -- Current Sensor (Three-Phase)/RConn1
  Phase Voltage Sensor (Three-Phase)/LConn1 -- Opabc/RConn1 -- RLC (Three-Phase)/RConn1

== system IndustrialMicrogrid/MG2 Primary Substation/BESS and Controller 2/BESS/Grid-Forming Converter Control ==
  Pref : Inport
  Qref : Inport  Port=2
  Vref : Inport  Port=3
  Fref : Inport  Port=4
  CntrlFlag : Inport  Port=5
  Igabc : Inport  Port=6
  Vgabc : Inport  Port=7
  BlackStart : Inport  Port=8
  Current Limiting : Subsystem
  Grid Voltage Reactive Power Support : Subsystem
  Measurement : Subsystem
      mask Display: image('$imagefile'); % Use "Edit Image" on toolstrip to change.
  Power Control : Subsystem
  VoltageCurrentControl : Subsystem
      settings: PortSchema="{\"entries\":[{\"content\":{\"sides\":[{\"content\":{\"connectorIds\":[\"In1\",\"In2\",\"In3\"]},\"type\":\"ConnectorPlacement.EquallySpacedRectSide\",\"uuid\":\"0bf15a12-7bc0-47e4-89bd-435769673763\"},{\"content\":{\"connectorIds\":[\"Out1\"],\"side\":\"RIGHT\"},\"type\":\"ConnectorPlacement.EquallySpacedRectSide\",\"uuid\":\"44a15d74-8878-4ec6-abe4-be0b1b609519\"},{\"content\":{\"connectorIds\":[\"In4\"],\"side\":\"TOP\"},\"type\":\"ConnectorPlacement.EquallySpacedRectSide\",\"uuid\":\"7a96781e-5638-4b2a-8101-d5785aae9f0f\"}]},\"type\":\"ConnectorPlacement.EquallySpacedConnector\",\"uuid\":\"4b3373ad-cf20-4175-894e-3bd1604dd0ce\"}],\"packageUris\":[\"http://schema.mathworks.com/mf0/Connector/R2020b\"],\"version\":\"1.0\"}"
  mabc : Outport
  Pmeas : Outport  Port=2
  Qmeas : Outport  Port=3
  fmeas : Outport  Port=4
  wires:
  VoltageCurrentControl/1(mabc) -> mabc/1
  Vgabc/1 -> Measurement/1(Vgabcc)
  Igabc/1 -> Measurement/2(Igabc)
  Measurement/2(Pmeas) -> Pmeas/1
  Measurement/3(Qmeas) -> Qmeas/1
  Measurement/1(measure) -> Current Limiting/1(measure), VoltageCurrentControl/4(measure), Power Control/1(measure), Grid Voltage Reactive Power Support/1(measure)
  Power Control/3(angle) -> Measurement/3(Angle)
  Power Control/1(reactiveControl) -> Current Limiting/2(reactiveControl)
  Power Control/2(activeControl) -> VoltageCurrentControl/2(activeControl)
  Current Limiting/1(currentLimiting) -> VoltageCurrentControl/1(currentLimiting)
  Qref/1 -> Grid Voltage Reactive Power Support/3(QrefInput)
  Pref/1 -> Grid Voltage Reactive Power Support/2(PrefInput)
  Grid Voltage Reactive Power Support/1(Pref) -> Power Control/2(Pref)
  Grid Voltage Reactive Power Support/2(Qref) -> Power Control/3(Qref)
  Measurement/4(fmeas) -> fmeas/1
  Fref/1 -> Power Control/5(Fref)
  Vref/1 -> Power Control/4(Vref)
  CntrlFlag/1 -> Power Control/6(CntrlFlag)
  BlackStart/1 -> VoltageCurrentControl/3(BlackStart)

== system IndustrialMicrogrid/MG2 Primary Substation/BESS and Controller 2/BESS/Per Unit Conversion ==
  fgrid : Inport
  Vabc : Inport  Port=2
  Iabc : Inport  Port=3
  Amp2PU : Gain  Gain=1/base.current
  PU2Hz : Gain  Gain=gridInverter.frequency
  Volt2PU : Gain  Gain=1/base.voltage
  fmeasHz : Outport
  Vabcpu : Outport  Port=2
  Iabcpu : Outport  Port=3
  wires:
  PU2Hz/1 -> fmeasHz/1
  fgrid/1 -> PU2Hz/1
  Volt2PU/1 -> Vabcpu/1  "Vabc"
  Iabc/1 -> Amp2PU/1
  Amp2PU/1 -> Iabcpu/1  "Iabc"
  Vabc/1 -> Volt2PU/1

== system IndustrialMicrogrid/MG2 Primary Substation/BESS and Controller 2/BESS/Subsystem ==
  PQref : Inport
  Demux : Demux  Outputs=2
  Low-Pass Filter (Discrete or Continuous) : eeGeneralControl/Low-Pass Filter (Discrete or Continuous)  K=1  T=5e-2  B=inf  A=-inf  init_option=Inherited from block input  x0=0  Ts=-1
  Low-Pass Filter (Discrete or Continuous)1 : eeGeneralControl/Low-Pass Filter (Discrete or Continuous)  K=1  T=5e-2  B=inf  A=-inf  init_option=Inherited from block input  x0=0  Ts=-1
  Unit Delay1 : UnitDelay  InitialCondition=1  SampleTime=Ts  HasFrameUpgradeWarning=on
  Unit Delay2 : UnitDelay  InitialCondition=1  SampleTime=Ts  HasFrameUpgradeWarning=on
  Pref : Outport
  Qref : Outport  Port=2
  wires:
  Demux/1 -> Unit Delay2/1  "Pref"
  Low-Pass Filter (Discrete or Continuous)/1 -> Pref/1
  Low-Pass Filter (Discrete or Continuous)1/1 -> Qref/1
  Demux/2 -> Unit Delay1/1  "Qref"
  PQref/1 -> Demux/1
  Unit Delay2/1 -> Low-Pass Filter (Discrete or Continuous)/1
  Unit Delay1/1 -> Low-Pass Filter (Discrete or Continuous)1/1

== system IndustrialMicrogrid/MG2 Primary Substation/BESS and Controller 2/BESS/Subsystem1 ==
  In1 : Inport
  Constant : Constant
  Constant1 : Constant  Value=0
  Switch : Switch  Criteria=u2 > Threshold  Threshold=0.5  SaturateOnIntegerOverflow=off  InputSameDT=off
  Out1 : Outport
  wires:
  Constant1/1 -> Switch/1
  Constant/1 -> Switch/3
  Switch/1 -> Out1/1
  In1/1 -> Switch/2

== system IndustrialMicrogrid/MG2 Primary Substation/BESS and Controller 2/BESS/Subsystem2 ==
  In1 : Inport
  In2 : Inport  Port=2
  AND : Logic  IconShape=distinctive  AllPortsSameDT=off  OutDataTypeStr=boolean
  Constant : Constant  Value=0
  Delay : Delay  DelayLength=microgrid.controller2BlackStartDelay  SampleTime=Ts*5000
  NOT : Logic  Operator=NOT  IconShape=distinctive  AllPortsSameDT=off  OutDataTypeStr=boolean
  Simulink-PS Converter : nesl_utility/Simulink-PS Converter  PhysicalDomain=network_engine_domain  SubClassName=ps_input  LeftPortType=input  RightPortType=output  PseudoPeriodic=off  Frequencies=[]  NoiseDistribution=none  NoiseParameters=[]  Unit=1  AffineConversion=off  FilteringAndDerivatives=provide  SimscapeFilterOrder=1  InputFilterTimeConstant=0.001  UdotUserProvided=0
  Switch : Switch  Criteria=u2 > Threshold  Threshold=0.5  SaturateOnIntegerOverflow=off  InputSameDT=off
  output : PMIOPort  Side=Right
  wires:
  AND/1 -> Switch/2
  Switch/1 -> Simulink-PS Converter/1
  In2/1 -> Switch/3
  In1/1 -> AND/1, Delay/1
  NOT/1 -> AND/2
  Constant/1 -> Switch/1
  Delay/1 -> NOT/1
  connections:
  Simulink-PS Converter/RConn1 -- output/RConn1

== system IndustrialMicrogrid/MG2 Primary Substation/BESS and Controller 2/BESS output filter and transformer1/Transformer 1 kV//13.8 kV ==
  "Transformer " : ee_lib/Passive/Transformers/Two-Winding Transformer (Three-Phase)  SRated=base.power*1e3 A*V  FRated=gridInverter.frequency Hz  Winding1Connection=ee.enum.windingconnection.Yg  VRated1=transformer.primaryRMSVoltage V  Winding2Connection=ee.enum.windingconnection.delta1  VRated2=transformer.secondaryRMSVoltage V  CoreType=ee.enum.coretype.threelimb  pu_Rw1=transformer.PrimaryResistancePU%*scrFactorRg  pu_Rw2=transformer.SecondaryResistancePU%*scrFactorRg  leakage_reactance_option=ee.enum.transformer_leakage.include  pu_Xl1=transformer.PrimaryReactancePU%*scrFactorXg  pu_Xl2=transformer.SecondaryReactancePU%*scrFactorXg  magnetizing_resistance_option=ee.enum.transformer_magnetizingResistance.exclude  pu_Rm=500  magnetizing_reactance_option=ee.enum.transformer_magnetizingReactance.exclude  saturation_option=ee.enum.transformer_saturation.exclude  pu_Xm=500  current_data=[0, .002, 1, 2]  magnetic_flux_data=[0, 1.2, 1.5, 1.51]  pu_X0=transformer.ZeroSequenceReactancePU%*scrFactorXg*1.1  i1_specify=on  i1_priority=None  i1=[0, 0, 0] A  i1_nominal_specify=off  i1_nominal_unit=A  i1_nominal_value=1  i2_specify=on  i2_priority=None  i2=[0, 0, 0] A  i2_nominal_specify=off  i2_nominal_unit=A  i2_nominal_value=1  phi_specify=off  phi_priority=None  phi=[0, 0, 0]  phi_nominal_specify=off  phi_nominal_unit=1  phi_nominal_value=1  power_dissipated_specify=off  power_dissipated_priority=None  power_dissipated=0 W  power_dissipated_nominal_specify=off  power_dissipated_nominal_unit=W  power_dissipated_nominal_value=1
      settings: InternalSimscapePortConfiguration="{\"Bottom\":[],\"Left\":[{\"id\":\"N1\",\"label\":\"~1\",\"type\":\"foundation.electrical.three_phase\"}],\"Right\":[{\"id\":\"N2\",\"label\":\"~2\",\"type\":\"foundation.electrical.three_phase\"}],\"Top\":[]}"
  ABC1 : PMIOPort  Side=Left
  ABC2 : PMIOPort  Port=2  Side=Right
  connections:
  "Transformer "/RConn1 -- ABC2/RConn1
  ABC1/RConn1 -- "Transformer "/LConn1

== system IndustrialMicrogrid/MG2 Primary Substation/Microgrid Controller 2/Black Start/If Action Subsystem ==
  Action Port : ActionPort  ActionPortLabel=if(u1 > 0)
  Constant : Constant  Value=60
  Subsystem : Subsystem
  Subsystem1 : Subsystem
  Subsystem2 : Subsystem
  Sum : Sum  Inputs=+++
  Out1 : Outport
  Out2 : Outport  Port=2
  wires:
  Constant/1 -> Out2/1
  Sum/1 -> Out1/1
  Subsystem2/1(Out1) -> Sum/1
  Subsystem/1(Out1) -> Sum/3
  Subsystem1/1(Out1) -> Sum/2

== system IndustrialMicrogrid/MG2 Primary Substation/Microgrid Controller 2/Black Start/If Action Subsystem1 ==
  Control Room : Inport
  Control Room1 : Inport  Port=2
  Action Port : ActionPort  ActionPortLabel=else
  Out1 : Outport
  Out2 : Outport  Port=2
  wires:
  Control Room/1 -> Out1/1
  Control Room1/1 -> Out2/1

== system IndustrialMicrogrid/MG2 Primary Substation/Microgrid Controller 2/PLL /PLL ==
  abc : Inport
  Rate Transition : RateTransition  Commented=through
  "Sinusoidal Measurement (PLL, Three-Phase)" : eeSinusoidalMeasurement/Sinusoidal Measurement (PLL, Three-Phase)  Kp_LF=KpPLLController2  Ki_LF=KIPLLController2  F0=GridFrequency  Theta0=0  Ts=Ts
  Subsystem : Subsystem
  fre : Outport
  angle : Outport  Port=2
  mag : Outport  Port=3
  wires:
  "Sinusoidal Measurement (PLL, Three-Phase)"/1 -> fre/1
  Subsystem/1(Out) -> angle/1
  "Sinusoidal Measurement (PLL, Three-Phase)"/2 -> Subsystem/1(In)
  Rate Transition/1 -> mag/1
  "Sinusoidal Measurement (PLL, Three-Phase)"/3 -> Rate Transition/1
  abc/1 -> "Sinusoidal Measurement (PLL, Three-Phase)"/1

== system IndustrialMicrogrid/MG2 Primary Substation/Microgrid Controller 2/PLL /PLL start at 0.2 s ==
  PCC measurement : Inport
  Constant : Constant  Value=0
  Step : Step  Time=0.2  SampleTime=Ts
  Switch : Switch  Criteria=u2 > Threshold  Threshold=0.5  SaturateOnIntegerOverflow=off  InputSameDT=off
  Out1 : Outport
  wires:
  Step/1 -> Switch/2
  Constant/1 -> Switch/3
  Switch/1 -> Out1/1
  PCC measurement/1 -> Switch/1

== system IndustrialMicrogrid/MG2 Primary Substation/Microgrid Controller 2/PLL /PLL starts at 0.2 s ==
  PCC measurement : Inport
  Constant1 : Constant  Value=0
  Step : Step  Time=0.2  SampleTime=Ts
  Switch : Switch  Criteria=u2 > Threshold  Threshold=0.5  SaturateOnIntegerOverflow=off  InputSameDT=off
  abc : Outport
  wires:
  Step/1 -> Switch/2
  Switch/1 -> abc/1
  Constant1/1 -> Switch/3
  PCC measurement/1 -> Switch/1

== system IndustrialMicrogrid/MG2 Primary Substation/Microgrid Controller 2/PLL /PLL1 ==
  abc : Inport
  "Sinusoidal Measurement (PLL, Three-Phase)" : eeSinusoidalMeasurement/Sinusoidal Measurement (PLL, Three-Phase)  Kp_LF=KpPLLController2  Ki_LF=KIPLLController2  F0=GridFrequency  Theta0=0  Ts=Ts
  Subsystem : Subsystem
  fre : Outport
  angle : Outport  Port=2
  mag : Outport  Port=3
  wires:
  abc/1 -> "Sinusoidal Measurement (PLL, Three-Phase)"/1
  "Sinusoidal Measurement (PLL, Three-Phase)"/3 -> mag/1
  "Sinusoidal Measurement (PLL, Three-Phase)"/2 -> Subsystem/1(In)
  Subsystem/1(Out) -> angle/1
  "Sinusoidal Measurement (PLL, Three-Phase)"/1 -> fre/1
